simulink model "lab4"  (R2018b)
settings: Solver=ode4  StartTime=0.0  StopTime=10  FixedStep=0.01  MaxStep=0.01  RelTol=1e-3
settings Model: Creator=Jakub  LastModifiedBy=PanLapek
settings SFSimCC: SimUseLocalCustomCode=off
settings RTWCC: RTWUseLocalCustomCode=off

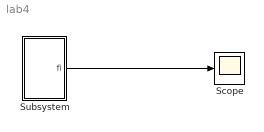
== system lab4 ==
  Scope : Scope
  Subsystem : Subsystem  mask{m=2, l=1, k=2, g=9.81, fi0=90}
      mask prompts: m "Masa"; l "Dlugosc"; fi0 "fi"
  wires:
  Subsystem/1("fi ") -> Scope/1

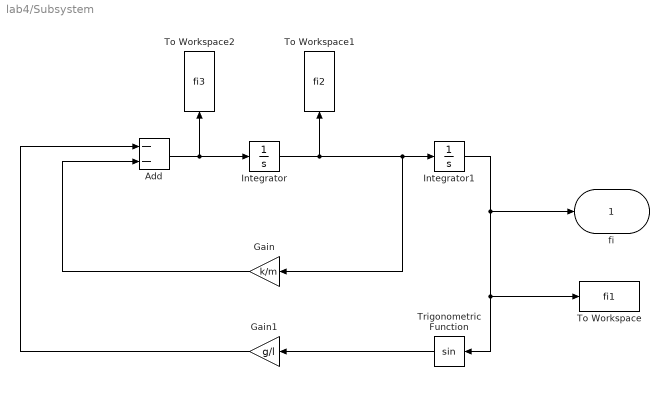
== system lab4/Subsystem ==
  Add : Sum  Inputs=--
  Gain : Gain  Gain=k/m
  Gain1 : Gain  Gain=g/l
  Integrator : Integrator
  Integrator1 : Integrator  InitialCondition=fi0*pi/180
  To Workspace : ToWorkspace  VariableName=fi1  SampleTime=-1
  To Workspace1 : ToWorkspace  VariableName=fi2  SampleTime=-1
  To Workspace2 : ToWorkspace  VariableName=fi3  SampleTime=-1
  Trigonometric Function : Trigonometry
  "fi " : Outport
  wires:
  Gain1/1 -> Add/1
  Gain/1 -> Add/2
  Integrator1/1 -> Trigonometric Function/1, To Workspace/1, "fi "/1
  Trigonometric Function/1 -> Gain1/1
  Integrator/1 -> Gain/1, Integrator1/1, To Workspace1/1
  Add/1 -> Integrator/1, To Workspace2/1
